simulink model "A1_MPC_AttitudeDynamics"  (R2017b)
settings: Solver=VariableStepAuto  StartTime=0.0  StopTime=20  FixedStep=1  MaxStep=0.1  RelTol=1e-6  EnableMultiTasking=on
StopFcn:
  | %attitudePlot = animateAttitude(rotmOut, 0.016);
  | %attitudePlot.plotInit;
  | %responsePlot(responseData, rotmOut, omegaRsOut, mechEnergyOut, mechPowerOut);
  | fprintf(2, 'max torque [mNm]: %5.2f', sqrt(max(torqueOut.Data(:,1).^2+torqueOut.Data(:,2).^2+torqueOut.Data(:,3).^2))*1000)
values from neighbouring files (symbols this model uses):
  J_sat = [2.5 2.5 2.5]    [AttitudeDynamicsData.m]
  T_disturb = ones(1,3) * 0.1E-3    [AttitudeDynamicsData.m]
undefined symbols (not defined in the file or in its folder): DiscIntNeverNeededParam, PID_MPC
libraries: SatelliteLibrary x15, mpclib x1, simulink x1
(part 1 of 2)
settings Model: Creator=Huib  LastModifiedBy=Huib
settings DataIOCC: LimitDataPoints=on
settings OptimizationCC: LifeSpan=inf
settings DebuggingCC: AllowSymbolicDim=off  SFUnexpectedBacktrackingDiag=warning  SFNoUnconditionalDefaultTransitionDiag=warning  SFExecutionAtInitializationDiag=none
settings ModelReferenceCC: PropagateSignalLabelsOutOfModel=off
settings CodeAppCC: StateflowObjectComments=on
settings GRTTargetCC: TargetLangStandard=C89/C90 (ANSI)
settings ConfigComp: CovMetricSettings=dw  CovHtmlReporting=on  CovSaveCumulativeToWorkspaceVar=on  CovSaveSingleToWorkspaceVar=on  CovExternalEMLEnable=off

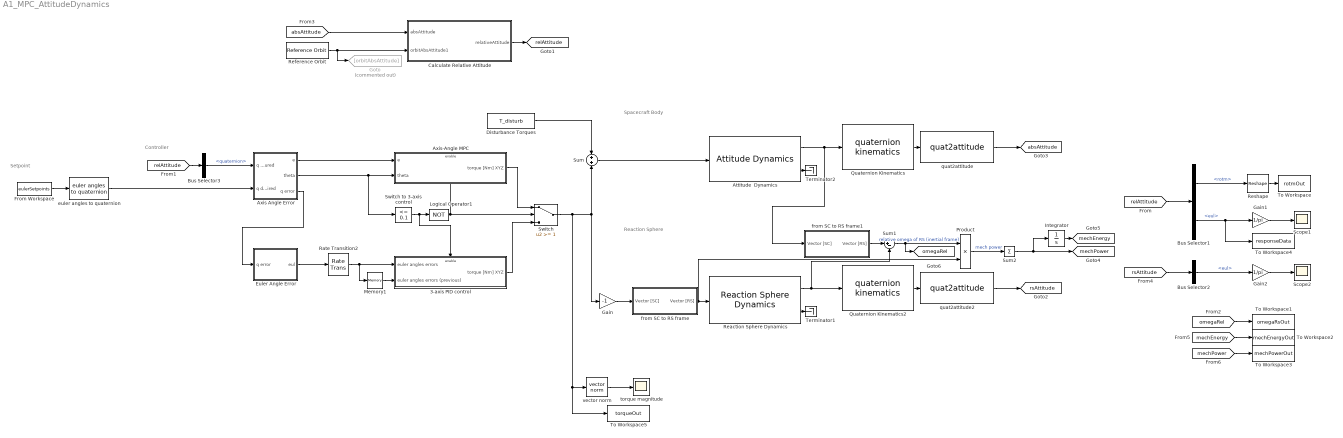
== system A1_MPC_AttitudeDynamics ==
  note: Setpoint
  note: Reaction Sphere
  note: Controller
  note: Spacecraft Body
  3-axis PID control : Subsystem
  Attitude  Dynamics : SatelliteLibrary/Attitude Dynamics  J11=J_sat(1)  J22=J_sat(2)  J33=J_sat(3)  omega0=w_zero
  Axis Angle Error : Subsystem
  Axis-Angle MPC : Subsystem
  Bus Selector1 : BusSelector  OutputSignals=rotm,eul
  Bus Selector2 : BusSelector  OutputSignals=eul
  Bus Selector3 : BusSelector  OutputSignals=quaternion
  Calculate Relative Attitude : Subsystem
  Disturbance Torques : Constant  Value=T_disturb
  Euler Angle Error : Subsystem
  From Workspace : FromWorkspace  VariableName=eulerSetpoints  SampleTime=0  Interpolate=off  OutputAfterFinalValue=Holding final value
  Gain : Gain  Gain=-1
  Gain1 : Gain  Gain=1/pi
  Gain2 : Gain  Gain=1/pi
  Goto : Goto  Commented=on  GotoTag=orbitAbsAttitude
  Integrator : Integrator
  Logical Operator1 : Logic  Operator=NOT  Inputs=1  AllPortsSameDT=off  OutDataTypeStr=boolean
  Memory1 : Memory
  Product : Product
  Quaternion Kinematics : SatelliteLibrary/quaternion kinematics  q_0=q_zero
  Quaternion Kinematics2 : SatelliteLibrary/quaternion kinematics  q_0=q_zero
  Rate Transition2 : RateTransition  OutPortSampleTime=0.1
  Reaction Sphere Dynamics : SatelliteLibrary/Reaction Sphere Dynamics  J=0.005567928416632  omega0=[0 0 0]
  Reference Orbit : SatelliteLibrary/Reference Orbit  orbitAltitude=700  gravParam=398600.4418  planetRadius=6371
  Reshape : Reshape  OutputDimensions=[9,1]
  Scope1 : Scope
  Scope2 : Scope
  Sum : Sum  Inputs=+|+
  Sum1 : Sum  Inputs=|+-
  Sum2 : Sum  Inputs=+
  Switch : Switch  Threshold=1
  Switch to 3-axis control : simulink/Logic and Bit Operations/Compare To Constant  relop=<=  const=0.1  OutDataTypeStr=boolean
  Terminator1 : Terminator
  Terminator2 : Terminator
  To Workspace : ToWorkspace  VariableName=rotmOut  SaveFormat=Timeseries  SampleTime=-1
  To Workspace1 : ToWorkspace  VariableName=omegaRsOut  SaveFormat=Timeseries  SampleTime=-1
  To Workspace2 : ToWorkspace  VariableName=mechEnergyOut  SaveFormat=Timeseries  SampleTime=-1
  To Workspace3 : ToWorkspace  VariableName=mechPowerOut  SaveFormat=Timeseries  SampleTime=-1
  To Workspace4 : ToWorkspace  VariableName=responseData  SaveFormat=Timeseries  SampleTime=-1
  To Workspace5 : ToWorkspace  VariableName=torqueOut  SaveFormat=Timeseries  SampleTime=-1
  euler angles to quaternion : SatelliteLibrary/euler angles to quaternion
  from SC to RS frame : Subsystem
  from SC to RS frame1 : Subsystem
  quat2attitude : SatelliteLibrary/quat2attitude
  quat2attitude2 : SatelliteLibrary/quat2attitude
  torque magnitude : Scope
  vector norm : SatelliteLibrary/vector norm
  tag scope: absAttitude=global, mechEnergy=global, mechPower=global, omegaRel=global, relAttitude=global, rsAttitude=global
  wires:
  Attitude  Dynamics/1 -> from SC to RS frame1/1(Vector [SC]), Quaternion Kinematics/1
  Quaternion Kinematics/1 -> quat2attitude/1
  Sum/1 -> Attitude  Dynamics/1
  Reshape/1 -> To Workspace/1
  Bus Selector1/1 -> Reshape/1  "<rotm>"
  Gain1/1 -> Scope1/1
  Sum1/1 -> [omegaRel], Product/1  "relative omega of RS (inertial frame)"
  Product/1 -> Sum2/1  "mech power"
  [absAttitude] -> Calculate Relative Attitude/1(absAttitude)
  Calculate Relative Attitude/1(relativeAttitude) -> [relAttitude]
  quat2attitude/1 -> [absAttitude]
  Reference Orbit/1 -> Goto/1, Calculate Relative Attitude/2(orbitAbsAttitude1)
  [relAttitude] -> Bus Selector3/1
  Disturbance Torques/1 -> Sum/1
  Switch/1 -> vector norm/1, To Workspace5/1, Gain/1, Sum/2
  [relAttitude] -> Bus Selector1/1
  Axis-Angle MPC/1(torque [Nm] XYZ) -> Switch/1
  Switch to 3-axis control/1 -> Logical Operator1/1, 3-axis PID control/Enable
  3-axis PID control/1(torque [Nm] XYZ) -> Switch/3
  From Workspace/1 -> euler angles to quaternion/1
  Logical Operator1/1 -> Switch/2, Axis-Angle MPC/Enable
  Rate Transition2/1 -> Memory1/1, 3-axis PID control/1(euler angles errors)
  Memory1/1 -> 3-axis PID control/2(euler angles errors (previous))
  [rsAttitude] -> Bus Selector2/1
  Bus Selector3/1 -> Axis Angle Error/1(q measured)  "<quaternion>"
  euler angles to quaternion/1 -> Axis Angle Error/2(q desired)
  Axis Angle Error/2(theta) -> Switch to 3-axis control/1, Axis-Angle MPC/2(theta)
  Axis Angle Error/1(e) -> Axis-Angle MPC/1(e)
  Axis Angle Error/3(q error) -> Euler Angle Error/1(q error)
  Euler Angle Error/1(eul) -> Rate Transition2/1
  Reaction Sphere Dynamics/1 -> Sum1/2, Quaternion Kinematics2/1
  Quaternion Kinematics2/1 -> quat2attitude2/1
  quat2attitude2/1 -> [rsAttitude]
  Gain/1 -> from SC to RS frame/1(Vector [SC])
  from SC to RS frame1/1(Vector [RS]) -> Sum1/1
  from SC to RS frame/1(Vector [RS]) -> Product/2, Reaction Sphere Dynamics/1
  Reaction Sphere Dynamics/2 -> Terminator1/1
  Attitude  Dynamics/2 -> Terminator2/1
  Bus Selector2/1 -> Gain2/1  "<eul>"
  Gain2/1 -> Scope2/1
  Integrator/1 -> [mechEnergy]
  Sum2/1 -> Integrator/1, [mechPower]
  [mechPower] -> To Workspace3/1
  [mechEnergy] -> To Workspace2/1
  [omegaRel] -> To Workspace1/1
  Bus Selector1/2 -> To Workspace4/1, Gain1/1  "<eul>"
  vector norm/1 -> torque magnitude/1

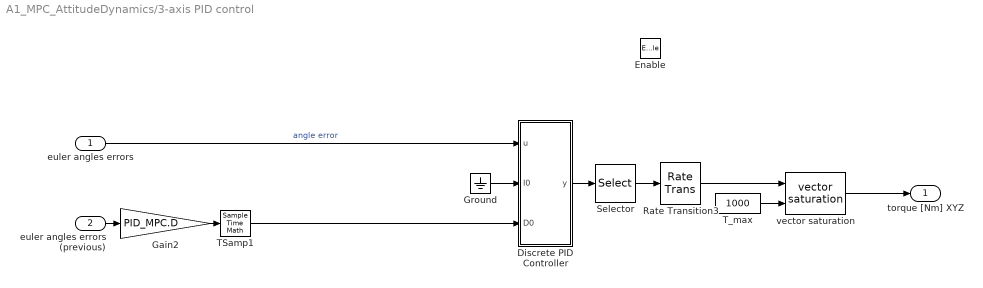
== system A1_MPC_AttitudeDynamics/3-axis PID control ==
  euler angles errors : Inport
  euler angles errors (previous) : Inport  Port=2
  Enable : EnablePort  StatesWhenEnabling=reset
  Discrete PID Controller : Subsystem  AncestorBlock=simulink/Continuous/PID Controller  DialogController=pidpack.PIDConfig.pidDDGCreate  mask(PID 1dof){Controller=PID, TimeDomain=Discrete-time, SampleTime=-1, IntegratorMethod=Forward Euler, FilterMethod=Forward Euler, Form=Parallel, UseFilter=off, ControllerParametersSource=internal, P=PID_MPC.P, I=PID_MPC.I, D=PID_MPC.D, N=1.14439525064094, InitialConditionSource=external, InitialConditionForIntegrator=0, InitialConditionForFilter=0, ExternalReset=none, IgnoreLimit=off, ZeroCross=on, LimitOutput=off, UpperSaturationLimit=inf, LowerSaturationLimit=-inf, LinearizeAsGain=off, AntiWindupMode=none, Kb=1, TrackingMode=off, Kt=1, RndMeth=Floor, SaturateOnIntegerOverflow=off, LockScale=off, PParamMin=[], PParamMax=[], PParamDataTypeStr=Inherit: Inherit via internal rule, IParamMin=[], IParamMax=[], IParamDataTypeStr=Inherit: Inherit via internal rule, DParamMin=[], DParamMax=[], DParamDataTypeStr=Inherit: Inherit via internal rule, NParamMin=[], NParamMax=[], NParamDataTypeStr=Inherit: Inherit via internal rule, KbParamMin=[], KbParamMax=[], KbParamDataTypeStr=Inherit: Inherit via internal rule, KtParamMin=[], KtParamMax=[], KtParamDataTypeStr=Inherit: Inherit via internal rule, POutMin=[], POutMax=[], POutDataTypeStr=Inherit: Inherit via internal rule, PGainOutDataTypeStr=Inherit: Inherit via internal rule, PProdOutDataTypeStr=Inherit: Inherit via internal rule, IOutMin=[], IOutMax=[], IOutDataTypeStr=Inherit: Inherit via internal rule, IGainOutDataTypeStr=Inherit: Inherit via internal rule, IProdOutDataTypeStr=Inherit: Inherit via internal rule, DOutMin=[], DOutMax=[], DOutDataTypeStr=Inherit: Inherit via internal rule, DGainOutDataTypeStr=Inherit: Inherit via internal rule, DProdOutDataTypeStr=Inherit: Inherit via internal rule, NOutMin=[], NOutMax=[], NOutDataTypeStr=Inherit: Inherit via internal rule, NGainOutDataTypeStr=Inherit: Inherit via internal rule, NProdOutDataTypeStr=Inherit: Inherit via internal rule, KbOutMin=[], KbOutMax=[], KbOutDataTypeStr=Inherit: Inherit via internal rule, KtOutMin=[], KtOutMax=[], KtOutDataTypeStr=Inherit: Inherit via internal rule, IntegratorOutMin=[], IntegratorOutMax=[], IntegratorOutDataTypeStr=Inherit: Inherit via internal rule, FilterOutMin=[], FilterOutMax=[], FilterOutDataTypeStr=Inherit: Inherit via internal rule, SumOutMin=[], SumOutMax=[], SumOutDataTypeStr=Inherit: Inherit via internal rule, SumI1OutMin=[], SumI1OutMax=[], SumI1OutDataTypeStr=Inherit: Inherit via internal rule, SumI2OutMin=[], SumI2OutMax=[], SumI2OutDataTypeStr=Inherit: Inherit via internal rule, SumI3OutMin=[], SumI3OutMax=[], SumI3OutDataTypeStr=Inherit: Inherit via internal rule, SumDOutMin=[], SumDOutMax=[], SumDOutDataTypeStr=Inherit: Inherit via internal rule, SumAccumDataTypeStr=Inherit: Inherit via internal rule, SumI1AccumDataTypeStr=Inherit: Inherit via internal rule, SumI2AccumDataTypeStr=Inherit: Inherit via internal rule, SumI3AccumDataTypeStr=Inherit: Inherit via internal rule, SumDAccumDataTypeStr=Inherit: Inherit via internal rule, SaturationOutMin=[], SaturationOutMax=[], SaturationOutDataTypeStr=Inherit: Same as input, IntegratorContinuousStateAttributes='', IntegratorStateIdentifier=, IntegratorStateMustResolveToSignalObject=off, IntegratorRTWStateStorageClass=Auto, IntegratorRTWStateStorageTypeQualifier=, FilterContinuousStateAttributes='', FilterStateIdentifier=, FilterStateMustResolveToSignalObject=off, FilterRTWStateStorageClass=Auto, FilterRTWStateStorageTypeQualifier=, DifferentiatorICPrevScaledInput=0, DifferentiatorOutMin=[], DifferentiatorOutMax=[], DifferentiatorOutDataTypeStr=Inherit: Inherit via internal rule, InitialConditionSetting=State (most efficient), FilterDiffNumProductOutputDataTypeStr=Inherit: Inherit via internal rule, FilterDiffDenProductOutputDataTypeStr=Inherit: Inherit via internal rule, FilterDiffNumAccumDataTypeStr=Inherit: Inherit via internal rule, FilterDiffDenAccumDataTypeStr=Inherit: Inherit via internal rule, FilterDiffOutCoefMin=[], FilterDiffOutCoefMax=[], FilterDiffOutCoefDataTypeStr=Inherit: Inherit via internal rule, SumDenAccumDataTypeStr=Inherit: Inherit via internal rule, SumDenOutMin=[], SumDenOutMax=[], SumDenOutDataTypeStr=Inherit: Inherit via internal rule, SumNumAccumDataTypeStr=Inherit: Inherit via internal rule, SumNumOutMin=[], SumNumOutMax=[], SumNumOutDataTypeStr=Inherit: Inherit via internal rule, ReciprocalOutMin=[], ReciprocalOutMax=[], ReciprocalOutDataTypeStr=Inherit: Inherit via internal rule, DivideOutMin=[], DivideOutMax=[], DivideOutDataTypeStr=Inherit: Inherit via internal rule, TunerSelectOption=Frequency Response Based}
      mask prompts: Controller "Simulink:masks:Controller_MP"; TimeDomain "Simulink:masks:TimeDomain_MP"; SampleTime "Simulink:masks:SampleTime1ForInherited_MP"; IntegratorMethod "Simulink:masks:IntegratorMethod_MP"; FilterMethod "Simulink:masks:FilterMethod_MP"; Form "Simulink:masks:Form_MP"; UseFilter "Simulink:masks:UseFilter_MP"; ControllerParametersSource "Simulink:masks:Source_MP"; P "Simulink:masks:ProportionalP_MP"; I "Simulink:masks:IntegralI_MP"; D "Simulink:masks:DerivativeD_MP"; N "Simulink:masks:FilterCoefficientN_MP"; InitialConditionSource "Simulink:masks:Source_MP"; InitialConditionForIntegrator "Simulink:masks:Integrator_MP"; InitialConditionForFilter "Simulink:masks:Filter_MP"; ExternalReset "Simulink:masks:ExternalReset_MP"; IgnoreLimit "Simulink:masks:IgnoreResetWhenLinearizing_MP"; ZeroCross "Simulink:masks:EnableZerocrossingDetection_MP"; LimitOutput "Simulink:masks:LimitOutput_MP"; UpperSaturationLimit "Simulink:masks:UpperSaturationLimit_MP"; LowerSaturationLimit "Simulink:masks:LowerSaturationLimit_MP"; LinearizeAsGain "Simulink:masks:IgnoreSaturationWhenLinearizing_MP"; AntiWindupMode "Simulink:masks:AntiwindupMethod_MP"; Kb "Simulink:masks:BackcalculationCoefficientKb_MP"; TrackingMode "Simulink:masks:EnableTrackingMode_MP"; Kt "Simulink:masks:TrackingCoefficientKt_MP"; RndMeth "Simulink:masks:IntegerRoundingMode_MP"; SaturateOnIntegerOverflow "Simulink:masks:SaturateOnIntegerOverflow_MP"; LockScale "Simulink:masks:LockDataTypeAgainstFxpTools_MP"; PParamMin "Simulink:masks:PParameterMinimum_MP"; PParamMax "Simulink:masks:PParameterMaximum_MP"; PParamDataTypeStr "Simulink:masks:PParameter_MP"; IParamMin "Simulink:masks:IParameterMinimum_MP"; IParamMax "Simulink:masks:IParameterMaximum_MP"; IParamDataTypeStr "Simulink:masks:IParameter_MP"; DParamMin "Simulink:masks:DParameterMinimum_MP"; DParamMax "Simulink:masks:DParameterMaximum_MP"; DParamDataTypeStr "Simulink:masks:DParameter_MP"; NParamMin "Simulink:masks:NParameterMinimum_MP"; NParamMax "Simulink:masks:NParameterMaximum_MP"; NParamDataTypeStr "Simulink:masks:NParameter_MP"; KbParamMin "Simulink:masks:KbParameterMinimum_MP"; KbParamMax "Simulink:masks:KbParameterMaximum_MP"; KbParamDataTypeStr "Simulink:masks:KbParameter_MP"; KtParamMin "Simulink:masks:KtParameterMinimum_MP"; KtParamMax "Simulink:masks:KtParameterMaximum_MP"; KtParamDataTypeStr "Simulink:masks:KtParameter_MP"; POutMin "Simulink:masks:PProductOutputMinimum_MP"; POutMax "Simulink:masks:PProductOutputMaximum_MP"; POutDataTypeStr "Simulink:masks:PProductOutput_MP"; PGainOutDataTypeStr "Simulink:masks:PProductOutput_MP"; PProdOutDataTypeStr "Simulink:masks:PProductOutput_MP"; IOutMin "Simulink:masks:IProductOutputMinimum_MP"; IOutMax "Simulink:masks:IProductOutputMaximum_MP"; IOutDataTypeStr "Simulink:masks:IProductOutput_MP"; IGainOutDataTypeStr "Simulink:masks:IProductOutput_MP"; IProdOutDataTypeStr "Simulink:masks:IProductOutput_MP"; DOutMin "Simulink:masks:DProductOutputMinimum_MP"; DOutMax "Simulink:masks:DProductOutputMaximum_MP"; DOutDataTypeStr "Simulink:masks:DProductOutput_MP"; DGainOutDataTypeStr "Simulink:masks:DProductOutput_MP"; DProdOutDataTypeStr "Simulink:masks:DProductOutput_MP"; NOutMin "Simulink:masks:NProductOutputMinimum_MP"; NOutMax "Simulink:masks:NProductOutputMaximum_MP"; NOutDataTypeStr "Simulink:masks:NProductOutput_MP"; NGainOutDataTypeStr "Simulink:masks:NProductOutput_MP"; NProdOutDataTypeStr "Simulink:masks:NProductOutput_MP"; KbOutMin "Simulink:masks:KbProductOutputMinimum_MP"; KbOutMax "Simulink:masks:KbProductOutputMaximum_MP"; KbOutDataTypeStr "Simulink:masks:KbProductOutput_MP"; KtOutMin "Simulink:masks:KtProductOutputMinimum_MP"; KtOutMax "Simulink:masks:KtProductOutputMaximum_MP"; KtOutDataTypeStr "Simulink:masks:KtProductOutput_MP"; IntegratorOutMin "Simulink:masks:IntegratorOutputMinimum_MP"; IntegratorOutMax "Simulink:masks:IntegratorOutputMaximum_MP"; IntegratorOutDataTypeStr "Simulink:masks:IntegratorOutput_MP"; FilterOutMin "Simulink:masks:FilterOutputMinimum_MP"; FilterOutMax "Simulink:masks:FilterOutputMaximum_MP"; FilterOutDataTypeStr "Simulink:masks:FilterOutput_MP"; SumOutMin "Simulink:masks:SumOutputMinimum_MP"; SumOutMax "Simulink:masks:SumOutputMaximum_MP"; SumOutDataTypeStr "Simulink:masks:SumOutput_MP"; SumI1OutMin "Simulink:masks:SumI1OutputMinimum_MP"; SumI1OutMax "Simulink:masks:SumI1OutputMaximum_MP"; SumI1OutDataTypeStr "Simulink:masks:SumI1Output_MP"; SumI2OutMin "Simulink:masks:SumI2OutputMinimum_MP"; SumI2OutMax "Simulink:masks:SumI2OutputMaximum_MP"; SumI2OutDataTypeStr "Simulink:masks:SumI2Output_MP"; SumI3OutMin "Simulink:masks:SumI3OutputMinimum_MP"; SumI3OutMax "Simulink:masks:SumI3OutputMaximum_MP"; SumI3OutDataTypeStr "Simulink:masks:SumI3Output_MP"; SumDOutMin "Simulink:masks:SumDOutputMinimum_MP"; SumDOutMax "Simulink:masks:SumDOutputMaximum_MP"; SumDOutDataTypeStr "Simulink:masks:SumDOutput_MP"; SumAccumDataTypeStr "Simulink:masks:AccumulatorOfSum_MP"; SumI1AccumDataTypeStr "Simulink:masks:AccumulatorOfSumI1_MP"; SumI2AccumDataTypeStr "Simulink:masks:AccumulatorOfSumI2_MP"; SumI3AccumDataTypeStr "Simulink:masks:AccumulatorOfSumI3_MP"; SumDAccumDataTypeStr "Simulink:masks:AccumulatorOfSumD_MP"; SaturationOutMin "Simulink:masks:SaturationOutputMinimum_MP"; SaturationOutMax "Simulink:masks:SaturationOutputMaximum_MP"; SaturationOutDataTypeStr "Simulink:masks:SaturationOutput_MP"; IntegratorContinuousStateAttributes "Simulink:masks:StateNameegposition_MP"; IntegratorStateIdentifier "Simulink:masks:StateName_MP"; IntegratorStateMustResolveToSignalObject "Simulink:masks:StateNameMustResolveToSimulinkSignalObject_MP"; IntegratorRTWStateStorageClass "Simulink:masks:CodeGenerationStorageClass_MP"; IntegratorRTWStateStorageTypeQualifier "Simulink:masks:CodeGenerationStorageTypeQualifier_MP"; FilterContinuousStateAttributes "Simulink:masks:StateNameegposition_MP"; FilterStateIdentifier "Simulink:masks:StateName_MP"; FilterStateMustResolveToSignalObject "Simulink:masks:StateNameMustResolveToSimulinkSignalObject_MP"; FilterRTWStateStorageClass "Simulink:masks:CodeGenerationStorageClass_MP"; FilterRTWStateStorageTypeQualifier "Simulink:masks:CodeGenerationStorageTypeQualifier_MP"; DifferentiatorICPrevScaledInput "Simulink:masks:Differentiator_MP"; DifferentiatorOutMin "Simulink:masks:DifferentiatorOutputMinimum_MP"; DifferentiatorOutMax "Simulink:masks:DifferentiatorOutputMaximum_MP"; DifferentiatorOutDataTypeStr "Simulink:masks:DifferentiatorOutput_MP"; InitialConditionSetting "Simulink:blkprm_prompts:IntegratorInitCondSetting"; FilterDiffNumProductOutputDataTypeStr "Simulink:masks:FilterDiffNumProductOutput_MP"; FilterDiffDenProductOutputDataTypeStr "Simulink:masks:FilterDiffDenProductOutput_MP"; FilterDiffNumAccumDataTypeStr "Simulink:masks:FilterDiffNumAccumulator_MP"; FilterDiffDenAccumDataTypeStr "Simulink:masks:FilterDiffDenAccumulator_MP"; FilterDiffOutCoefMin "Simulink:masks:FilterDiffCoefficientOutputMinimum_MP"; FilterDiffOutCoefMax "Simulink:masks:FilterDiffCoefficientOutputMaximum_MP"; FilterDiffOutCoefDataTypeStr "Simulink:masks:FilterDiffCoefficientOutput_MP"; SumDenAccumDataTypeStr "Simulink:masks:FilterDiffSumDenAccumulator_MP"; SumDenOutMin "Simulink:masks:FilterDiffSumDenOutputMinimum_MP"; SumDenOutMax "Simulink:masks:FilterDiffSumDenOutputMaximum_MP"; SumDenOutDataTypeStr "Simulink:masks:FilterDiffSumDenOutput_MP"; SumNumAccumDataTypeStr "Simulink:masks:FilterDiffSumNumAccumulator_MP"; SumNumOutMin "Simulink:masks:FilterDiffSumNumOutputMinimum_MP"; SumNumOutMax "Simulink:masks:FilterDiffSumNumOutputMaximum_MP"; SumNumOutDataTypeStr "Simulink:masks:FilterDiffSumNumOutput_MP"; ReciprocalOutMin "Simulink:masks:FilterDiffReciprocalOutputMinimum_MP"; ReciprocalOutMax "Simulink:masks:FilterDiffReciprocalOutputMaximum_MP"; ReciprocalOutDataTypeStr "Simulink:masks:FilterDiffReciprocalOutput_MP"; DivideOutMin "Simulink:masks:FilterDiffDivideOutputMinimum_MP"; DivideOutMax "Simulink:masks:FilterDiffDivideOutputMaximum_MP"; DivideOutDataTypeStr "Simulink:masks:FilterDiffDivideOutput_MP"; TunerSelectOption "Simulink:masks:PIDAutoTuningMethodSelect_MP"
      mask help: Simulink:masks:PID1dof_MD
      mask init:
      | pidpack.PIDConfig.configPID(gcbh);
      settings: DeleteFcn=pidpack.PIDConfig.closeTuner(gcbh)  ModelCloseFcn=pidpack.PIDConfig.closeTuner(gcbh)  NameChangeFcn=pidpack.PIDConfig.updateTunerName(gcbh)
      mask TypeOptions Controller: Simulink:masks:PID | Simulink:masks:PI | Simulink:masks:PD | Simulink:masks:P | Simulink:masks:I
      mask TypeOptions TimeDomain: Simulink:masks:ContinuousTime | Simulink:masks:DiscreteTime
      mask TypeOptions SampleTime: u/SampleTime | y/SampleTime | r/SampleTime | RESET/SampleTime | I0/SampleTime | D0/SampleTime | TR/SampleTime | Clamping circuit/preSat/SampleTime | Clamping circuit/preIntegrator/SampleTime | Clamping circuit/preP/SampleTime | Clamping circuit/AND/SampleTime | Clamping circuit/AND1/SampleTime | Clamping circuit/AND2/SampleTime | Clamping circuit/AND3/SampleTime | Clamping circuit/Gain/SampleTime | Clamping circuit/DataTypeConv2/SampleTime | Clamping circuit/DataTypeConv3/SampleTime | Clamping circuit/DeadZone/SampleTime | Clamping circuit/Equal/SampleTime | Clamping circuit/Equal1/SampleTime | Clamping circuit/Equal2/SampleTime | Clamping circuit/NOT1/SampleTime | Clamping circuit/NOT2/SampleTime | Clamping circuit/NotEqual/SampleTime | Clamping circuit/OR1/SampleTime | Clamping circuit/SignPreIntegrator/SampleTime | Clamping circuit/SignPreP/SampleTime | Clamping circuit/SignPreSat/SampleTime | Clamping circuit/Clamp/SampleTime | Derivative Gain/SampleTime | Filter/SampleTime | Filter Coefficient/SampleTime | Integral Gain/SampleTime | Integrator/SampleTime | Kb/SampleTime | Kt/SampleTime | Proportional Gain/SampleTime | Saturate/SampleTime | sprintf('/Setpoint Weighting\n(Derivative)')/SampleTime | sprintf('/Setpoint Weighting\n(Proportional)')/SampleTime | Sum/SampleTime | Sum1/SampleTime | Sum2/SampleTime | Sum3/SampleTime | SumD/SampleTime | SumI1/SampleTime | SumI2/SampleTime | SumI3/SampleTime | Switch/SampleTime | Differentiator/U/SampleTime | Differentiator/Y/SampleTime | POut/SampleTime | IOut/SampleTime | DOut/SampleTime | NOut/SampleTime | P/SampleTime | I/SampleTime | D/SampleTime | N/SampleTime | Proportional Gain Fdbk/SampleTime | Saturate Fdbk/SampleTime | Sum Fdbk/SampleTime | POut Fdbk/SampleTime | Filter Differentiator/Constant/SampleTime | Filter Differentiator/DenCoefOut/SampleTime | Filter Differentiator/Divide/SampleTime | Filter Differentiator/Filter Differentiator TF/SampleTime | Filter Differentiator/N/SampleTime | Filter Differentiator/NOut/SampleTime | Filter Differentiator/Reciprocal/SampleTime | Filter Differentiator/SumDen/SampleTime | Filter Differentiator/SumNum/SampleTime | Filter Differentiator/Unary Minus/SampleTime | P Copy/SampleTime | Filter Differentiator/RESET/SampleTime | Filter Differentiator/D0/SampleTime | Filter Differentiator/Filter Coefficient/SampleTime | Filter Differentiator/U/SampleTime | Filter Differentiator/Y/SampleTime
      mask TypeOptions IntegratorMethod: Simulink:masks:ForwardEuler | Simulink:masks:BackwardEuler | Simulink:masks:Trapezoidal
      mask TypeOptions FilterMethod: Simulink:masks:ForwardEuler | Simulink:masks:BackwardEuler | Simulink:masks:Trapezoidal
      mask TypeOptions Form: Simulink:masks:Ideal | Simulink:masks:Parallel
      mask TypeOptions ControllerParametersSource: Simulink:masks:internal | Simulink:masks:external
      mask TypeOptions P: Proportional Gain/Gain | Proportional Gain Fdbk/Gain | P Copy/Value
      mask TypeOptions I: Integral Gain/Gain
      mask TypeOptions D: Derivative Gain/Gain
      mask TypeOptions N: Filter Coefficient/Gain | Filter Differentiator/Filter Coefficient/Gain | Filter Differentiator/N Copy/Value
      mask TypeOptions InitialConditionSource: Simulink:masks:internal | Simulink:masks:external
      mask TypeOptions InitialConditionForIntegrator: Integrator/InitialCondition
      mask TypeOptions InitialConditionForFilter: Filter/InitialCondition | Filter Differentiator/Filter Differentiator TF/InitialStates
      mask TypeOptions ExternalReset: Simulink:masks:none | Simulink:masks:rising | Simulink:masks:falling | Simulink:masks:either | Simulink:masks:level
      mask TypeOptions UpperSaturationLimit: Clamping circuit/DeadZone/UpperValue | Saturate/UpperLimit | Saturate Fdbk/UpperLimit
      mask TypeOptions LowerSaturationLimit: Clamping circuit/DeadZone/LowerValue | Saturate/LowerLimit | Saturate Fdbk/LowerLimit
      mask TypeOptions AntiWindupMode: Simulink:masks:none | Simulink:masks:backCalculation | Simulink:masks:clamping
      mask TypeOptions Kb: Kb/Gain
      mask TypeOptions Kt: Kt/Gain
      mask TypeOptions RndMeth: Clamping circuit/Gain/RndMeth | Clamping circuit/DataTypeConv2/RndMeth | Clamping circuit/DataTypeConv3/RndMeth | Derivative Gain/RndMeth | Differentiator/RndMeth | Filter/RndMeth | Filter Coefficient/RndMeth | Integral Gain/RndMeth | Integrator/RndMeth | Kb/RndMeth | Kt/RndMeth | Proportional Gain/RndMeth | Saturate/RndMeth | sprintf('/Setpoint Weighting\n(Derivative)')/RndMeth | sprintf('/Setpoint Weighting\n(Proportional)')/RndMeth | Sum/RndMeth | Sum1/RndMeth | Sum2/RndMeth | Sum3/RndMeth | SumD/RndMeth | SumI1/RndMeth | SumI2/RndMeth | SumI3/RndMeth | Switch/RndMeth | Differentiator/TSamp/RndMeth | Differentiator/Diff/RndMeth | POut/RndMeth | IOut/RndMeth | DOut/RndMeth | NOut/RndMeth | Proportional Gain Fdbk/RndMeth | Saturate Fdbk/RndMeth | Sum Fdbk/RndMeth | POut Fdbk/RndMeth | Filter Differentiator/DenCoefOut/RndMeth | Filter Differentiator/Divide/RndMeth | Filter Differentiator/Filter Differentiator TF/RndMeth | Filter Differentiator/NOut/RndMeth | Filter Differentiator/Reciprocal/RndMeth | Filter Differentiator/SumDen/RndMeth | Filter Differentiator/SumNum/RndMeth | Filter Differentiator/TSamp/RndMeth | Filter Differentiator/Filter Coefficient/RndMeth
      mask TypeOptions SaturateOnIntegerOverflow: Clamping circuit/Gain/SaturateOnIntegerOverflow | Clamping circuit/DataTypeConv2/SaturateOnIntegerOverflow | Clamping circuit/DataTypeConv3/SaturateOnIntegerOverflow | Clamping circuit/DeadZone/SaturateOnIntegerOverflow | Derivative Gain/SaturateOnIntegerOverflow | Filter/SaturateOnIntegerOverflow | Filter Coefficient/SaturateOnIntegerOverflow | Integral Gain/SaturateOnIntegerOverflow | Integrator/SaturateOnIntegerOverflow | Kb/SaturateOnIntegerOverflow | Kt/SaturateOnIntegerOverflow | Proportional Gain/SaturateOnIntegerOverflow | sprintf('/Setpoint Weighting\n(Derivative)')/SaturateOnIntegerOverflow | sprintf('/Setpoint Weighting\n(Proportional)')/SaturateOnIntegerOverflow | Sum/SaturateOnIntegerOverflow | Sum1/SaturateOnIntegerOverflow | Sum2/SaturateOnIntegerOverflow | Sum3/SaturateOnIntegerOverflow | SumD/SaturateOnIntegerOverflow | SumI1/SaturateOnIntegerOverflow | SumI2/SaturateOnIntegerOverflow | SumI3/SaturateOnIntegerOverflow | Switch/SaturateOnIntegerOverflow | Differentiator/TSamp/SaturateOnIntegerOverflow | Differentiator/Diff/SaturateOnIntegerOverflow | POut/SaturateOnIntegerOverflow | IOut/SaturateOnIntegerOverflow | DOut/SaturateOnIntegerOverflow | NOut/SaturateOnIntegerOverflow | Proportional Gain Fdbk/SaturateOnIntegerOverflow | Sum Fdbk/SaturateOnIntegerOverflow | POut Fdbk/SaturateOnIntegerOverflow | Filter Differentiator/DenCoefOut/SaturateOnIntegerOverflow | Filter Differentiator/Divide/SaturateOnIntegerOverflow | Filter Differentiator/Filter Differentiator TF/SaturateOnIntegerOverflow | Filter Differentiator/NOut/SaturateOnIntegerOverflow | Filter Differentiator/Reciprocal/SaturateOnIntegerOverflow | Filter Differentiator/SumDen/SaturateOnIntegerOverflow | Filter Differentiator/SumNum/SaturateOnIntegerOverflow | Filter Differentiator/TSamp/SaturateOnIntegerOverflow | Filter Differentiator/Unary Minus/SaturateOnIntegerOverflow | Filter Differentiator/Filter Coefficient/SaturateOnIntegerOverflow
      mask TypeOptions LockScale: Clamping circuit/preSat/LockScale | Clamping circuit/preIntegrator/LockScale | Clamping circuit/preP/LockScale | Clamping circuit/Gain/LockScale | Clamping circuit/DataTypeConv2/LockScale | Clamping circuit/DataTypeConv3/LockScale | Clamping circuit/Clamp/LockScale | Constant/LockScale | Derivative Gain/LockScale | Differentiator/LockScale | Filter/LockScale | Filter Coefficient/LockScale | Integral Gain/LockScale | Integrator/LockScale | Kb/LockScale | Kt/LockScale | Proportional Gain/LockScale | Saturate/LockScale | sprintf('/Setpoint Weighting\n(Derivative)')/LockScale | sprintf('/Setpoint Weighting\n(Proportional)')/LockScale | Sum/LockScale | Sum1/LockScale | Sum2/LockScale | Sum3/LockScale | SumD/LockScale | SumI1/LockScale | SumI2/LockScale | SumI3/LockScale | Switch/LockScale | Differentiator/U/LockScale | Differentiator/Diff/LockScale | Differentiator/Y/LockScale | POut/LockScale | IOut/LockScale | DOut/LockScale | NOut/LockScale | Proportional Gain Fdbk/LockScale | Saturate Fdbk/LockScale | Sum Fdbk/LockScale | POut Fdbk/LockScale | Filter Differentiator/Constant/LockScale | Filter Differentiator/DenCoefOut/LockScale | Filter Differentiator/Divide/LockScale | Filter Differentiator/Filter Differentiator TF/LockScale | Filter Differentiator/N/LockScale | Filter Differentiator/NOut/LockScale | Filter Differentiator/Reciprocal/LockScale | Filter Differentiator/SumDen/LockScale | Filter Differentiator/SumNum/LockScale | P Copy/LockScale | Filter Differentiator/Filter Coefficient/LockScale | Filter Differentiator/U/LockScale | Filter Differentiator/Y/LockScale
      mask TypeOptions PParamMin: Proportional Gain/ParamMin | Proportional Gain Fdbk/ParamMin | P Copy/OutMin
      mask TypeOptions PParamMax: Proportional Gain/ParamMax | Proportional Gain Fdbk/ParamMax | P Copy/OutMax
      mask TypeOptions PParamDataTypeStr: Proportional Gain/ParamDataTypeStr | Proportional Gain Fdbk/ParamDataTypeStr
      mask TypeOptions IParamMin: Integral Gain/ParamMin
      mask TypeOptions IParamMax: Integral Gain/ParamMax
      mask TypeOptions IParamDataTypeStr: Integral Gain/ParamDataTypeStr
      mask TypeOptions DParamMin: Derivative Gain/ParamMin
      mask TypeOptions DParamMax: Derivative Gain/ParamMax
      mask TypeOptions DParamDataTypeStr: Derivative Gain/ParamDataTypeStr
      mask TypeOptions NParamMin: Filter Coefficient/ParamMin | Filter Differentiator/Filter Coefficient/ParamMin | Filter Differentiator/N Copy/OutMin
      mask TypeOptions NParamMax: Filter Coefficient/ParamMax | Filter Differentiator/Filter Coefficient/ParamMax | Filter Differentiator/N Copy/OutMax
      mask TypeOptions NParamDataTypeStr: Filter Coefficient/ParamDataTypeStr | Filter Differentiator/Filter Coefficient/ParamDataTypeStr
      mask TypeOptions KbParamMin: Kb/ParamMin
      mask TypeOptions KbParamMax: Kb/ParamMax
      mask TypeOptions KbParamDataTypeStr: Kb/ParamDataTypeStr
      mask TypeOptions KtParamMin: Kt/ParamMin
      mask TypeOptions KtParamMax: Kt/ParamMax
      mask TypeOptions KtParamDataTypeStr: Kt/ParamDataTypeStr
      mask TypeOptions POutMin: Proportional Gain/OutMin | POut/OutMin | Proportional Gain Fdbk/OutMin | POut Fdbk/OutMin
      mask TypeOptions POutMax: Proportional Gain/OutMax | POut/OutMax | Proportional Gain Fdbk/OutMax | POut Fdbk/OutMax
      mask TypeOptions PGainOutDataTypeStr: Proportional Gain/OutDataTypeStr | Proportional Gain Fdbk/OutDataTypeStr
      mask TypeOptions PProdOutDataTypeStr: POut/OutDataTypeStr | POut Fdbk/OutDataTypeStr
      mask TypeOptions IOutMin: Integral Gain/OutMin | IOut/OutMin
      mask TypeOptions IOutMax: Integral Gain/OutMax | IOut/OutMax
      mask TypeOptions IGainOutDataTypeStr: Integral Gain/OutDataTypeStr
      mask TypeOptions IProdOutDataTypeStr: IOut/OutDataTypeStr
      mask TypeOptions DOutMin: Derivative Gain/OutMin | DOut/OutMin
      mask TypeOptions DOutMax: Derivative Gain/OutMax | DOut/OutMax
      mask TypeOptions DGainOutDataTypeStr: Derivative Gain/OutDataTypeStr
      mask TypeOptions DProdOutDataTypeStr: DOut/OutDataTypeStr
      mask TypeOptions NOutMin: Filter Coefficient/OutMin | NOut/OutMin | Filter Differentiator/Filter Coefficient/OutMin | Filter Differentiator/NOut/OutMin
      mask TypeOptions NOutMax: Filter Coefficient/OutMax | NOut/OutMax | Filter Differentiator/Filter Coefficient/OutMax | Filter Differentiator/NOut/OutMax
      mask TypeOptions NGainOutDataTypeStr: Filter Coefficient/OutDataTypeStr | Filter Differentiator/Filter Coefficient/OutDataTypeStr
      mask TypeOptions NProdOutDataTypeStr: NOut/OutDataTypeStr | Filter Differentiator/NOut/OutDataTypeStr
      mask TypeOptions KbOutMin: Kb/OutMin
      mask TypeOptions KbOutMax: Kb/OutMax
      mask TypeOptions KbOutDataTypeStr: Kb/OutDataTypeStr
      mask TypeOptions KtOutMin: Kt/OutMin
      mask TypeOptions KtOutMax: Kt/OutMax
      mask TypeOptions KtOutDataTypeStr: Kt/OutDataTypeStr
      mask TypeOptions IntegratorOutMin: Integrator/OutMin
      mask TypeOptions IntegratorOutMax: Integrator/OutMax
      mask TypeOptions IntegratorOutDataTypeStr: Integrator/OutDataTypeStr
      mask TypeOptions FilterOutMin: Filter/OutMin
      mask TypeOptions FilterOutMax: Filter/OutMax
      mask TypeOptions FilterOutDataTypeStr: Filter/OutDataTypeStr
      mask TypeOptions SumOutMin: Sum/OutMin | Sum Fdbk/OutMin
      mask TypeOptions SumOutMax: Sum/OutMax | Sum Fdbk/OutMax
      mask TypeOptions SumOutDataTypeStr: Sum/OutDataTypeStr | Sum Fdbk/OutDataTypeStr
      mask TypeOptions SumI1OutMin: SumI1/OutMin
      mask TypeOptions SumI1OutMax: SumI1/OutMax
      mask TypeOptions SumI1OutDataTypeStr: SumI1/OutDataTypeStr
      mask TypeOptions SumI2OutMin: SumI2/OutMin
      mask TypeOptions SumI2OutMax: SumI2/OutMax
      mask TypeOptions SumI2OutDataTypeStr: SumI2/OutDataTypeStr
      mask TypeOptions SumI3OutMin: SumI3/OutMin
      mask TypeOptions SumI3OutMax: SumI3/OutMax
      mask TypeOptions SumI3OutDataTypeStr: SumI3/OutDataTypeStr
      mask TypeOptions SumDOutMin: SumD/OutMin
      mask TypeOptions SumDOutMax: SumD/OutMax
      mask TypeOptions SumDOutDataTypeStr: SumD/OutDataTypeStr
      mask TypeOptions SumAccumDataTypeStr: Sum/AccumDataTypeStr | Sum Fdbk/AccumDataTypeStr
      mask TypeOptions SumI1AccumDataTypeStr: SumI1/AccumDataTypeStr
      mask TypeOptions SumI2AccumDataTypeStr: SumI2/AccumDataTypeStr
      mask TypeOptions SumI3AccumDataTypeStr: SumI3/AccumDataTypeStr
      mask TypeOptions SumDAccumDataTypeStr: SumD/AccumDataTypeStr
      mask TypeOptions SaturationOutMin: Saturate/OutMin | Saturate Fdbk/OutMin
      mask TypeOptions SaturationOutMax: Saturate/OutMax | Saturate Fdbk/OutMax
      mask TypeOptions SaturationOutDataTypeStr: Saturate/OutDataTypeStr | Saturate Fdbk/OutDataTypeStr
      mask TypeOptions IntegratorContinuousStateAttributes: Integrator/ContinuousStateAttributes
      mask TypeOptions IntegratorStateIdentifier: Integrator/StateIdentifier
      mask TypeOptions IntegratorRTWStateStorageClass: Simulink:masks:Auto | Simulink:masks:ExportedGlobal | Simulink:masks:ImportedExtern | Simulink:masks:ImportedExternPointer
      mask TypeOptions FilterContinuousStateAttributes: Filter/ContinuousStateAttributes
      mask TypeOptions FilterStateIdentifier: Filter/StateIdentifier | Filter Differentiator/Filter Differentiator TF/StateIdentifier
      mask TypeOptions FilterRTWStateStorageClass: Simulink:masks:Auto | Simulink:masks:ExportedGlobal | Simulink:masks:ImportedExtern | Simulink:masks:ImportedExternPointer
      mask TypeOptions DifferentiatorICPrevScaledInput: Differentiator/UD/InitialCondition
      mask TypeOptions InitialConditionSetting: Integrator/InitialConditionSetting | Filter/InitialConditionSetting
      mask TypeOptions FilterDiffNumProductOutputDataTypeStr: Filter Differentiator/Filter Differentiator TF/NumProductDataTypeStr
      mask TypeOptions FilterDiffDenProductOutputDataTypeStr: Filter Differentiator/Filter Differentiator TF/DenProductDataTypeStr
      mask TypeOptions FilterDiffNumAccumDataTypeStr: Filter Differentiator/Filter Differentiator TF/NumAccumDataTypeStr
      mask TypeOptions FilterDiffDenAccumDataTypeStr: Filter Differentiator/Filter Differentiator TF/DenAccumDataTypeStr
      mask TypeOptions FilterDiffOutCoefMin: Filter Differentiator/DenCoefOut/OutMin
      mask TypeOptions FilterDiffOutCoefMax: Filter Differentiator/DenCoefOut/OutMax
      mask TypeOptions FilterDiffOutCoefDataTypeStr: Filter Differentiator/DenCoefOut/OutDataTypeStr
      mask TypeOptions SumDenAccumDataTypeStr: Filter Differentiator/SumDen/AccumDataTypeStr
      mask TypeOptions SumDenOutMin: Filter Differentiator/SumDen/OutMin
      mask TypeOptions SumDenOutMax: Filter Differentiator/SumDen/OutMax
      mask TypeOptions SumDenOutDataTypeStr: Filter Differentiator/SumDen/OutDataTypeStr
      mask TypeOptions SumNumAccumDataTypeStr: Filter Differentiator/SumNum/AccumDataTypeStr
      mask TypeOptions SumNumOutMin: Filter Differentiator/SumNum/OutMin
      mask TypeOptions SumNumOutMax: Filter Differentiator/SumNum/OutMax
      mask TypeOptions SumNumOutDataTypeStr: Filter Differentiator/SumNum/OutDataTypeStr
      mask TypeOptions ReciprocalOutMin: Filter Differentiator/Reciprocal/OutMin
      mask TypeOptions ReciprocalOutMax: Filter Differentiator/Reciprocal/OutMax
      mask TypeOptions ReciprocalOutDataTypeStr: Filter Differentiator/Reciprocal/OutDataTypeStr
      mask TypeOptions DivideOutMin: Filter Differentiator/Divide/OutMin
      mask TypeOptions DivideOutMax: Filter Differentiator/Divide/OutMax
      mask TypeOptions DivideOutDataTypeStr: Filter Differentiator/Divide/OutDataTypeStr
      mask TypeOptions TunerSelectOption: Simulink:masks:UsePIDTunerApp | Simulink:masks:UseOLSimulation
      mask DialogControl Controller Prompt: Controller:
      mask DialogControl TimeDomain Prompt: Time domain:
      mask DialogControl SampleTime Prompt: Sample time (-1 for inherited):
      mask DialogControl IntegratorMethod Prompt: Integrator method:
      mask DialogControl FilterMethod Prompt: Filter method:
      mask DialogControl Form Prompt: Form:
      mask DialogControl UseFilter Prompt: Use filtered derivative
      mask DialogControl ControllerParametersSource Prompt: Source:
      mask DialogControl P Prompt: Proportional (P):
      mask DialogControl I Prompt: Integral (I):
      mask DialogControl D Prompt: Derivative (D):
      mask DialogControl N Prompt: Filter coefficient (N):
      mask DialogControl InitialConditionSource Prompt: Source:
      mask DialogControl InitialConditionForIntegrator Prompt: Integrator:
      mask DialogControl InitialConditionForFilter Prompt: Filter:
      mask DialogControl ExternalReset Prompt: External reset:
      mask DialogControl IgnoreLimit Prompt: Ignore reset when linearizing
      mask DialogControl ZeroCross Prompt: Enable zero-crossing detection
      mask DialogControl LimitOutput Prompt: Limit output
      mask DialogControl UpperSaturationLimit Prompt: Upper saturation limit:
      mask DialogControl LowerSaturationLimit Prompt: Lower saturation limit:
      mask DialogControl LinearizeAsGain Prompt: Ignore saturation when linearizing
      mask DialogControl AntiWindupMode Prompt: Anti-windup method:
      mask DialogControl Kb Prompt: Back-calculation coefficient (Kb):
      mask DialogControl TrackingMode Prompt: Enable tracking mode
      mask DialogControl Kt Prompt: Tracking coefficient (Kt):
      mask DialogControl RndMeth Prompt: Integer rounding mode:
      mask DialogControl SaturateOnIntegerOverflow Prompt: Saturate on integer overflow
      mask DialogControl LockScale Prompt: Lock data type settings against changes by the fixed-point tools
      mask DialogControl PParamMin Prompt: P parameter minimum:
      mask DialogControl PParamMax Prompt: P parameter maximum:
      mask DialogControl PParamDataTypeStr Prompt: P parameter:
      mask DialogControl IParamMin Prompt: I parameter minimum:
      mask DialogControl IParamMax Prompt: I parameter maximum:
      mask DialogControl IParamDataTypeStr Prompt: I parameter:
      mask DialogControl DParamMin Prompt: D parameter minimum:
      mask DialogControl DParamMax Prompt: D parameter maximum:
      mask DialogControl DParamDataTypeStr Prompt: D parameter:
      mask DialogControl NParamMin Prompt: N parameter minimum:
      mask DialogControl NParamMax Prompt: N parameter maximum:
      mask DialogControl NParamDataTypeStr Prompt: N parameter:
      mask DialogControl KbParamMin Prompt: Kb parameter minimum:
      mask DialogControl KbParamMax Prompt: Kb parameter maximum:
      mask DialogControl KbParamDataTypeStr Prompt: Kb parameter:
      mask DialogControl KtParamMin Prompt: Kt parameter minimum:
      mask DialogControl KtParamMax Prompt: Kt parameter maximum:
      mask DialogControl KtParamDataTypeStr Prompt: Kt parameter:
      mask DialogControl POutMin Prompt: P product output minimum:
      mask DialogControl POutMax Prompt: P product output maximum:
      mask DialogControl POutDataTypeStr Prompt: P product output:
      mask DialogControl PGainOutDataTypeStr Prompt: P product output:
      mask DialogControl PProdOutDataTypeStr Prompt: P product output:
      mask DialogControl IOutMin Prompt: I product output minimum:
      mask DialogControl IOutMax Prompt: I product output maximum:
      mask DialogControl IOutDataTypeStr Prompt: I product output:
      mask DialogControl IGainOutDataTypeStr Prompt: I product output:
      mask DialogControl IProdOutDataTypeStr Prompt: I product output:
      mask DialogControl DOutMin Prompt: D product output minimum:
      mask DialogControl DOutMax Prompt: D product output maximum:
      mask DialogControl DOutDataTypeStr Prompt: D product output:
      mask DialogControl DGainOutDataTypeStr Prompt: D product output:
      mask DialogControl DProdOutDataTypeStr Prompt: D product output:
      mask DialogControl NOutMin Prompt: N product output minimum:
      mask DialogControl NOutMax Prompt: N product output maximum:
      mask DialogControl NOutDataTypeStr Prompt: N product output:
      mask DialogControl NGainOutDataTypeStr Prompt: N product output:
      mask DialogControl NProdOutDataTypeStr Prompt: N product output:
      mask DialogControl KbOutMin Prompt: Kb product output minimum:
      mask DialogControl KbOutMax Prompt: Kb product output maximum:
      mask DialogControl KbOutDataTypeStr Prompt: Kb product output:
      mask DialogControl KtOutMin Prompt: Kt product output minimum:
      mask DialogControl KtOutMax Prompt: Kt product output maximum:
      mask DialogControl KtOutDataTypeStr Prompt: Kt product output:
      mask DialogControl IntegratorOutMin Prompt: Integrator output minimum:
      mask DialogControl IntegratorOutMax Prompt: Integrator output maximum:
      mask DialogControl IntegratorOutDataTypeStr Prompt: Integrator output:
      mask DialogControl FilterOutMin Prompt: Filter output minimum:
      mask DialogControl FilterOutMax Prompt: Filter output maximum:
      mask DialogControl FilterOutDataTypeStr Prompt: Filter output:
      mask DialogControl SumOutMin Prompt: Sum output minimum:
      mask DialogControl SumOutMax Prompt: Sum output maximum:
      mask DialogControl SumOutDataTypeStr Prompt: Sum output:
      mask DialogControl SumI1OutMin Prompt: SumI1 output minimum:
      mask DialogControl SumI1OutMax Prompt: SumI1 output maximum:
      mask DialogControl SumI1OutDataTypeStr Prompt: SumI1 output:
      mask DialogControl SumI2OutMin Prompt: SumI2 output minimum:
      mask DialogControl SumI2OutMax Prompt: SumI2 output maximum:
      mask DialogControl SumI2OutDataTypeStr Prompt: SumI2 output:
      mask DialogControl SumI3OutMin Prompt: SumI3 output minimum:
      mask DialogControl SumI3OutMax Prompt: SumI3 output maximum:
      mask DialogControl SumI3OutDataTypeStr Prompt: SumI3 output:
      mask DialogControl SumDOutMin Prompt: SumD output minimum:
      mask DialogControl SumDOutMax Prompt: SumD output maximum:
      mask DialogControl SumDOutDataTypeStr Prompt: SumD output:
      mask DialogControl SumAccumDataTypeStr Prompt: Accumulator of Sum:
      mask DialogControl SumI1AccumDataTypeStr Prompt: Accumulator of SumI1:
      mask DialogControl SumI2AccumDataTypeStr Prompt: Accumulator of SumI2:
      mask DialogControl SumI3AccumDataTypeStr Prompt: Accumulator of SumI3:
      mask DialogControl SumDAccumDataTypeStr Prompt: Accumulator of SumD:
      mask DialogControl SaturationOutMin Prompt: Saturation output minimum:
      mask DialogControl SaturationOutMax Prompt: Saturation output maximum:
      mask DialogControl SaturationOutDataTypeStr Prompt: Saturation output:
      mask DialogControl IntegratorContinuousStateAttributes Prompt: State name: (e.g., 'position')
      mask DialogControl IntegratorStateIdentifier Prompt: State name:
      mask DialogControl IntegratorStateMustResolveToSignalObject Prompt: State name must resolve to Simulink signal object
      mask DialogControl IntegratorRTWStateStorageClass Prompt: Code generation storage class:
      mask DialogControl IntegratorRTWStateStorageTypeQualifier Prompt: Code generation storage type qualifier:
      mask DialogControl FilterContinuousStateAttributes Prompt: State name: (e.g., 'position')
      mask DialogControl FilterStateIdentifier Prompt: State name:
      mask DialogControl FilterStateMustResolveToSignalObject Prompt: State name must resolve to Simulink signal object
      mask DialogControl FilterRTWStateStorageClass Prompt: Code generation storage class:
      mask DialogControl FilterRTWStateStorageTypeQualifier Prompt: Code generation storage type qualifier:
      mask DialogControl DifferentiatorICPrevScaledInput Prompt: Differentiator:
      mask DialogControl DifferentiatorOutMin Prompt: Differentiator output minimum:
      mask DialogControl DifferentiatorOutMax Prompt: Differentiator output maximum:
      mask DialogControl DifferentiatorOutDataTypeStr Prompt: Differentiator output:
      mask DialogControl InitialConditionSetting Prompt: Initial condition setting:
      mask DialogControl FilterDiffNumProductOutputDataTypeStr Prompt: Filter Numerator product output:
      mask DialogControl FilterDiffDenProductOutputDataTypeStr Prompt: Filter Denominator product output:
      mask DialogControl FilterDiffNumAccumDataTypeStr Prompt: Filter Numerator accumulator:
      mask DialogControl FilterDiffDenAccumDataTypeStr Prompt: Filter Denominator accumulator:
      mask DialogControl FilterDiffOutCoefMin Prompt: Filter Coefficient product output minimum:
      mask DialogControl FilterDiffOutCoefMax Prompt: Filter Coefficient product output maximum:
      mask DialogControl FilterDiffOutCoefDataTypeStr Prompt: Filter Coefficient product output:
      mask DialogControl SumDenAccumDataTypeStr Prompt: Accumulator of SumDen:
      mask DialogControl SumDenOutMin Prompt: SumDen output minimum:
      mask DialogControl SumDenOutMax Prompt: SumDen output maximum:
      mask DialogControl SumDenOutDataTypeStr Prompt: SumDen output:
      mask DialogControl SumNumAccumDataTypeStr Prompt: Accumulator of SumNum:
      mask DialogControl SumNumOutMin Prompt: SumNum output minimum:
      mask DialogControl SumNumOutMax Prompt: SumNum output maximum:
      mask DialogControl SumNumOutDataTypeStr Prompt: SumNum output:
      mask DialogControl ReciprocalOutMin Prompt: Reciprocal output minimum:
      mask DialogControl ReciprocalOutMax Prompt: Reciprocal output maximum:
      mask DialogControl ReciprocalOutDataTypeStr Prompt: Reciprocal output:
      mask DialogControl DivideOutMin Prompt: Divide output minimum:
      mask DialogControl DivideOutMax Prompt: Divide output maximum:
      mask DialogControl DivideOutDataTypeStr Prompt: Divide output:
      mask DialogControl TunerSelectOption Prompt: Select Tuning Method:
      mask Display:
      | iconstr = pidpack.PIDConfig.getMaskDisplayString(gcbh);
      | eval(iconstr)
  Gain2 : Gain  Gain=PID_MPC.D
  Ground : Ground
  Rate Transition3 : RateTransition
  Selector : Selector  InputPortWidth=3  IndexOptions=Index vector (dialog)  Indices=[3 2 1]  OutputSizes=1
  TSamp1 : SampleTimeMath  TsampMathOp=/  TsampMathImp=Offline Scaling Adjustment
  T_max : Constant  Value=1000
  vector saturation : SatelliteLibrary/vector saturation
  torque [Nm] XYZ : Outport
  wires:
  euler angles errors/1 -> Discrete PID Controller/1(u)  "angle error"
  T_max/1 -> vector saturation/2
  Selector/1 -> Rate Transition3/1
  Rate Transition3/1 -> vector saturation/1
  vector saturation/1 -> torque [Nm] XYZ/1
  Discrete PID Controller/1(y) -> Selector/1
  Ground/1 -> Discrete PID Controller/2(I0)
  euler angles errors (previous)/1 -> Gain2/1
  TSamp1/1 -> Discrete PID Controller/3(D0)
  Gain2/1 -> TSamp1/1

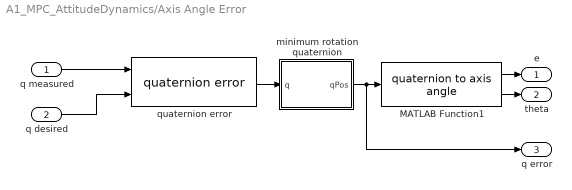
== system A1_MPC_AttitudeDynamics/Axis Angle Error ==
  q measured : Inport
  q desired : Inport  Port=2
  MATLAB Function1 : SatelliteLibrary/quaternion to axis angle
  minimum rotation quaternion : MATLAB Function  TreatAsAtomicUnit=on
  quaternion error : SatelliteLibrary/quaternion error
  e : Outport
  theta : Outport  Port=2
  q error : Outport  Port=3
  wires:
  q desired/1 -> quaternion error/2
  MATLAB Function1/1 -> e/1
  quaternion error/1 -> minimum rotation quaternion/1(q)
  minimum rotation quaternion/1(qPos) -> q error/1, MATLAB Function1/1
  MATLAB Function1/2 -> theta/1
  q measured/1 -> quaternion error/1
